simulink model "abssq06_fixpt16"  (R2021b)
settings: Solver=VariableStepAuto  StartTime=0.0  StopTime=99  RelTol=1e-3
undefined symbols (not defined in the file): S, vsva2197, xcvc1902
libraries: hdlBasic x65, vmcUtilities x1
settings Model: Creator=abeshu  LastModifiedBy=shu_abe

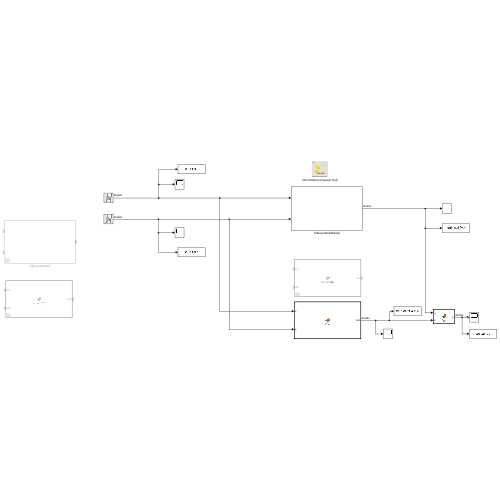
[thumbnail: Simulink's stored preview of the top-level diagram]
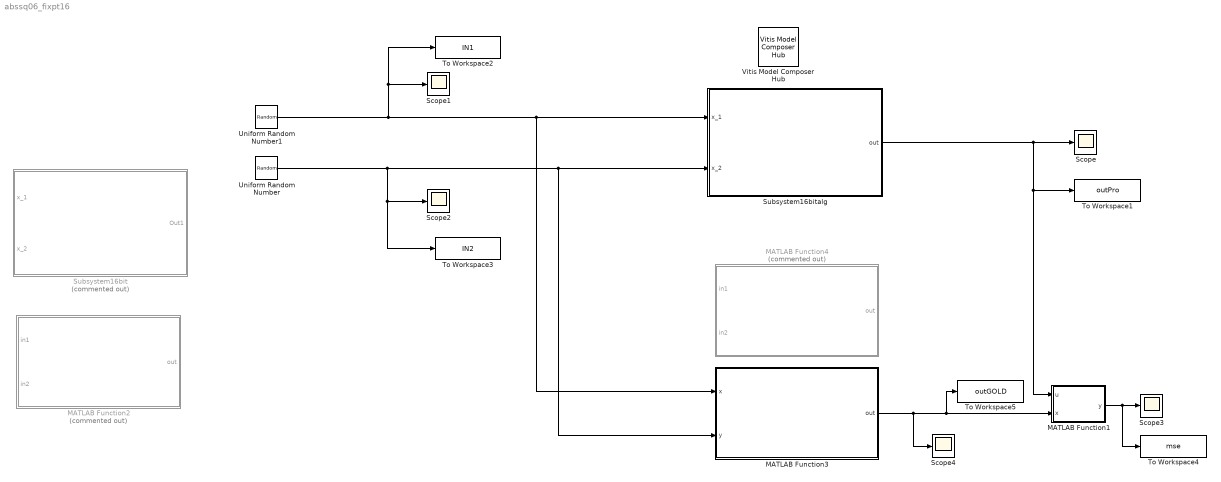
== system abssq06_fixpt16 ==
  MATLAB Function1 : MATLAB Function  TreatAsAtomicUnit=on
  MATLAB Function2 : MATLAB Function  Commented=on  TreatAsAtomicUnit=on
  MATLAB Function3 : MATLAB Function  TreatAsAtomicUnit=on
  MATLAB Function4 : MATLAB Function  Commented=on  TreatAsAtomicUnit=on
  Scope{,1..4} (5 alike) : Scope
  Subsystem16bit : Subsystem  Commented=on
      mask Display: %%%%
  Subsystem16bitalg : Subsystem
      mask Display: %%%%
  To Workspace1 : ToWorkspace  VariableName=outPro  SaveFormat=Structure With Time  SampleTime=-1
  To Workspace2 : ToWorkspace  VariableName=IN1  SaveFormat=Structure With Time  SampleTime=-1
  To Workspace3 : ToWorkspace  VariableName=IN2  SaveFormat=Structure With Time  SampleTime=-1
  To Workspace4 : ToWorkspace  VariableName=mse  SaveFormat=Structure With Time  SampleTime=-1
  To Workspace5 : ToWorkspace  VariableName=outGOLD  SaveFormat=Structure With Time  SampleTime=-1
  Uniform Random Number : UniformRandomNumber  SampleTime=1
  Uniform Random Number1 : UniformRandomNumber  Seed=1  SampleTime=1
  Vitis Model Composer Hub : vmcUtilities/Vitis Model Composer Hub  Tag=genX  CodeGeneration=off  SubsystemName=<enter or select subsystem name>  TargetDirectory=./code  ExportType=HLS C++ code  IpVendor=xilinx.com  IpLibrary=hls  IpVersion=1.0  IpHWLanguage=Verilog  AieCompilerOptions={}  CreateTestbench=off  TestbenchStackSize=10  RunAieSim=off  AieSimTimeout=50000  RunAieSimProfiling=off  LaunchVitisAnalyzer=off  PlotOutput=off  RunX86Sim=off  X86SimTimeout=10  GenHwImage=off  PlatformType=Not Specified  HwSystemType=Baremetal  HwValidationTarget=hw  ProjDevice=Alveo U250 Data Center Accelerator Card (xcu250-figd2104-2L-e)  ProjDevicePart=xcvc1902-vsva2197-2MP-e-S  SamplePeriod=-1  ClockFrequency=200  DataPathParallelism=1  xilinxfamily=virtexuplus  part=xcu250  speed=-2L-e  package=figd2104  directory=./abssq06alg_sim16  testbench=on  incr_netlist=off  synthesis_tool=Vivado  clock_wrapper=Clock Enables  dbl_ovrd=According to Block Masks  dcm_input_clock_period=10  sysclk_period=50  simulink_period=1  eval_field=0
  wires:
  Subsystem16bitalg/1(out) -> Scope/1, MATLAB Function1/1(u), To Workspace1/1
  MATLAB Function1/1(y) -> To Workspace4/1, Scope3/1
  MATLAB Function3/1(out) -> Scope4/1, To Workspace5/1, MATLAB Function1/2(x)
  Uniform Random Number1/1 -> Subsystem16bitalg/1(x_1), MATLAB Function3/1(x), To Workspace2/1, Scope1/1
  Uniform Random Number/1 -> Subsystem16bitalg/2(x_2), MATLAB Function3/2(y), To Workspace3/1, Scope2/1

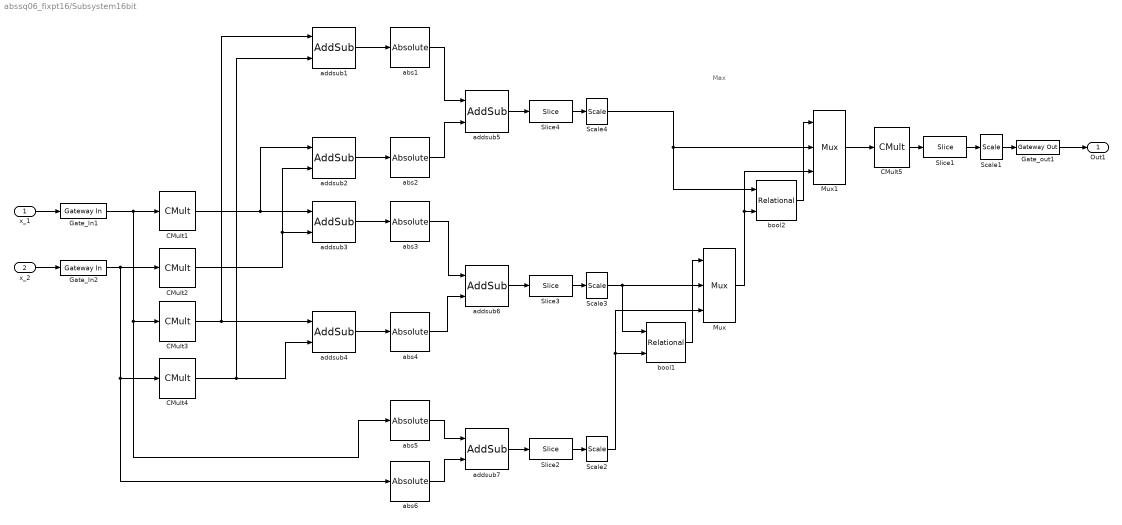
== system abssq06_fixpt16/Subsystem16bit ==
  note: Max
  x_1 : Inport
  x_2 : Inport  Port=2
  CMult1 : hdlBasic/CMult  const=cos(pi/6)  gui_display_data_type=Fixed-point  const_n_bits=16  const_bin_pt=15  float_type=Single  exp_bits=8  fraction_bits=24  en=off  latency=0  precision=Full  arith_type="Signed  (2's comp)"  n_bits=16  bin_pt=14  quantization=Truncate  overflow=Wrap  use_behavioral_HDL=off  mem_type=Distributed RAM  pipeline=off  XmcBlockStatus=1  maskContainerNames=tabcontainer1  block_type=cmult  block_config=sysgen:CMult_config
      settings: infoedit=[]
  CMult2 : hdlBasic/CMult  const=sin(pi/6)  gui_display_data_type=Fixed-point  const_n_bits=16  const_bin_pt=15  float_type=Single  exp_bits=8  fraction_bits=24  en=off  latency=0  precision=Full  arith_type="Signed  (2's comp)"  n_bits=16  bin_pt=14  quantization=Truncate  overflow=Wrap  use_behavioral_HDL=off  mem_type=Distributed RAM  pipeline=off  XmcBlockStatus=1  maskContainerNames=tabcontainer1  block_type=cmult  block_config=sysgen:CMult_config
      settings: infoedit=[]
  CMult3 : hdlBasic/CMult  const=sin(pi/6)  gui_display_data_type=Fixed-point  const_n_bits=16  const_bin_pt=15  float_type=Single  exp_bits=8  fraction_bits=24  en=off  latency=0  precision=Full  arith_type="Signed  (2's comp)"  n_bits=16  bin_pt=14  quantization=Truncate  overflow=Wrap  use_behavioral_HDL=off  mem_type=Distributed RAM  pipeline=off  XmcBlockStatus=1  maskContainerNames=tabcontainer1  block_type=cmult  block_config=sysgen:CMult_config
      settings: infoedit=[]
  CMult4 : hdlBasic/CMult  const=cos(pi/6)  gui_display_data_type=Fixed-point  const_n_bits=16  const_bin_pt=15  float_type=Single  exp_bits=8  fraction_bits=24  en=off  latency=0  precision=Full  arith_type="Signed  (2's comp)"  n_bits=16  bin_pt=14  quantization=Truncate  overflow=Wrap  use_behavioral_HDL=off  mem_type=Distributed RAM  pipeline=off  XmcBlockStatus=1  maskContainerNames=tabcontainer1  block_type=cmult  block_config=sysgen:CMult_config
      settings: infoedit=[]
  CMult5 : hdlBasic/CMult  const=1/sqrt(2)  gui_display_data_type=Fixed-point  const_n_bits=16  const_bin_pt=15  float_type=Single  exp_bits=8  fraction_bits=24  en=off  latency=0  precision=Full  arith_type="Signed  (2's comp)"  n_bits=16  bin_pt=14  quantization=Truncate  overflow=Wrap  use_behavioral_HDL=off  mem_type=Distributed RAM  pipeline=off  XmcBlockStatus=1  maskContainerNames=tabcontainer1  block_type=cmult  block_config=sysgen:CMult_config
      settings: infoedit=[]
  Gate_In1 : hdlBasic/Gateway In  gui_display_data_type=Fixed-point  arith_type=Signed (2's comp)  n_bits=16  bin_pt=14  preci_type=Double  exp_width=8  frac_width=24  rows=1  columns=1  quantization="Round  (unbiased: +/- Inf)"  overflow=Saturate  period=1  UseAsADC=off  ADCChannel='1'  interface=None  automatic_assignment=on  address_offset=hex2dec('00')  intf_name=''  intf_description=''  default_value=0  timing_constraint=None  locs_specified=off  LOCs={}  io_standard={}  inherit_from_input=off  hdl_port=on  XmcBlockStatus=1  maskContainerNames=group4  block_type=gatewayin  block_config=sysgen:gateway_in_config  block_width_w=590  block_height_w=620  block_width=640  block_height=850
  Gate_In2 : hdlBasic/Gateway In  gui_display_data_type=Fixed-point  arith_type=Signed (2's comp)  n_bits=16  bin_pt=14  preci_type=Double  exp_width=8  frac_width=24  rows=1  columns=1  quantization="Round  (unbiased: +/- Inf)"  overflow=Saturate  period=1  UseAsADC=off  ADCChannel='1'  interface=None  automatic_assignment=on  address_offset=hex2dec('00')  intf_name=''  intf_description=''  default_value=0  timing_constraint=None  locs_specified=off  LOCs={}  io_standard={}  inherit_from_input=off  hdl_port=on  XmcBlockStatus=1  maskContainerNames=group4  block_type=gatewayin  block_config=sysgen:gateway_in_config  block_width_w=590  block_height_w=620  block_width=640  block_height=850
  Gate_out1 : hdlBasic/Gateway Out  inherit_from_input=off  hdl_port=on  rows=1  columns=1  UseAsDAC=off  DACChannel='1'  interface=None  automatic_assignment=on  address_offset=hex2dec('00')  intf_name=''  intf_description=''  timing_constraint=None  locs_specified=off  LOCs={}  io_standard={}  XmcBlockStatus=1  maskContainerNames=group4  block_type=gatewayout  block_config=sysgen:gateway_out_config  block_width_w=590  block_height_w=620  block_width=620  block_height=750
  Mux : hdlBasic/Mux  inputs=2  en=off  latency=0  precision=Full  arith_type=Unsigned  n_bits=16  bin_pt=14  quantization=Truncate  overflow=Wrap  XmcBlockStatus=1  maskContainerNames=tabcontainer1  block_type=mux  block_config=sysgen:Mux_config
  Mux1 : hdlBasic/Mux  inputs=2  en=off  latency=0  precision=Full  arith_type=Unsigned  n_bits=16  bin_pt=14  quantization=Truncate  overflow=Wrap  XmcBlockStatus=1  maskContainerNames=tabcontainer1  block_type=mux  block_config=sysgen:Mux_config
  Scale1 : hdlBasic/Scale  scale_factor=-15  XmcBlockStatus=1  maskContainerNames=group1  block_type=scale  block_config=sysgen:Scale_config
  Scale2 : hdlBasic/Scale  scale_factor=-14  XmcBlockStatus=1  maskContainerNames=group1  block_type=scale  block_config=sysgen:Scale_config
  Scale3 : hdlBasic/Scale  scale_factor=-15  XmcBlockStatus=1  maskContainerNames=group1  block_type=scale  block_config=sysgen:Scale_config
  Scale4 : hdlBasic/Scale  scale_factor=-15  XmcBlockStatus=1  maskContainerNames=group1  block_type=scale  block_config=sysgen:Scale_config
  Slice1 : hdlBasic/Slice  nbits=8  boolean_output=off  mode=Two Bit Locations  bit1=-1  base1=MSB of Input  bit0=15  base0=LSB of Input  XmcBlockStatus=1  maskContainerNames=group1  block_type=slice  block_config=sysgen:Slice_config
  Slice2 : hdlBasic/Slice  nbits=15  boolean_output=off  mode=Upper Bit Location + Width  bit1=-3  base1=MSB of Input  bit0=7  base0=LSB of Input  XmcBlockStatus=1  maskContainerNames=group1  block_type=slice  block_config=sysgen:Slice_config
  Slice3 : hdlBasic/Slice  nbits=7  boolean_output=off  mode=Two Bit Locations  bit1=-5  base1=MSB of Input  bit0=14  base0=LSB of Input  XmcBlockStatus=1  maskContainerNames=group1  block_type=slice  block_config=sysgen:Slice_config
  Slice4 : hdlBasic/Slice  nbits=7  boolean_output=off  mode=Two Bit Locations  bit1=-5  base1=MSB of Input  bit0=14  base0=LSB of Input  XmcBlockStatus=1  maskContainerNames=group1  block_type=slice  block_config=sysgen:Slice_config
  abs{1..6} (6 alike) : hdlBasic/Absolute  precision=Full  arith_type=Unsigned  n_bits=16  bin_pt=14  quantization=Truncate  overflow=Wrap  en=off  latency=0  XmcBlockStatus=1  maskContainerNames=tabcontainer1  block_type=abs  block_config=sysgen:Abs_config
  addsub1 : hdlBasic/AddSub  mode=Subtraction  use_carryin=off  use_carryout=off  en=off  latency=0  precision=Full  arith_type="Signed  (2's comp)"  n_bits=35  bin_pt=32  quantization="Round  (unbiased: +/- Inf)"  overflow=Saturate  use_behavioral_HDL=off  hw_selection=Fabric  pipelined=on  XmcBlockStatus=1  maskContainerNames=tabcontainer1  block_type=addsub  block_config=sysgen:Addsub_config
  addsub{2,4..6} (4 alike) : hdlBasic/AddSub  mode=Addition  use_carryin=off  use_carryout=off  en=off  latency=0  precision=Full  arith_type=Unsigned  n_bits=16  bin_pt=14  quantization="Round  (unbiased: +/- Inf)"  overflow=Saturate  use_behavioral_HDL=off  hw_selection=Fabric  pipelined=on  XmcBlockStatus=1  maskContainerNames=tabcontainer1  block_type=addsub  block_config=sysgen:Addsub_config
  addsub3 : hdlBasic/AddSub  mode=Subtraction  use_carryin=off  use_carryout=off  en=off  latency=0  precision=Full  arith_type="Signed  (2's comp)"  n_bits=35  bin_pt=32  quantization="Round  (unbiased: +/- Inf)"  overflow=Saturate  use_behavioral_HDL=off  hw_selection=Fabric  pipelined=on  XmcBlockStatus=1  maskContainerNames=tabcontainer1  block_type=addsub  block_config=sysgen:Addsub_config
  addsub7 : hdlBasic/AddSub  mode=Addition  use_carryin=off  use_carryout=off  en=off  latency=0  precision=Full  arith_type=Unsigned  n_bits=17  bin_pt=16  quantization="Round  (unbiased: +/- Inf)"  overflow=Saturate  use_behavioral_HDL=off  hw_selection=Fabric  pipelined=on  XmcBlockStatus=1  maskContainerNames=tabcontainer1  block_type=addsub  block_config=sysgen:Addsub_config
  bool1 : hdlBasic/Relational  mode=a<b  op_type=Bool  en=off  latency=0  XmcBlockStatus=1  maskContainerNames=tabcontainer1  block_type=relational  block_config=sysgen:Relational_config
  bool2 : hdlBasic/Relational  mode=a<b  op_type=Bool  en=off  latency=0  XmcBlockStatus=1  maskContainerNames=tabcontainer1  block_type=relational  block_config=sysgen:Relational_config
  Out1 : Outport
  wires:
  addsub3/1 -> abs3/1
  abs3/1 -> addsub6/1
  CMult1/1 -> addsub3/1, addsub2/1
  CMult2/1 -> addsub3/2, addsub2/2
  CMult5/1 -> Slice1/1
  x_2/1 -> Gate_In2/1
  x_1/1 -> Gate_In1/1
  bool1/1 -> Mux/1
  addsub4/1 -> abs4/1
  abs4/1 -> addsub6/2
  Gate_In1/1 -> CMult1/1, abs5/1, CMult3/1
  Gate_In2/1 -> CMult4/1, abs6/1, CMult2/1
  CMult3/1 -> addsub4/1, addsub1/1
  CMult4/1 -> addsub4/2, addsub1/2
  addsub2/1 -> abs2/1
  abs2/1 -> addsub5/2
  addsub1/1 -> abs1/1
  abs1/1 -> addsub5/1
  Gate_out1/1 -> Out1/1
  Scale4/1 -> bool2/1, Mux1/2
  Mux/1 -> Mux1/3, bool2/2
  bool2/1 -> Mux1/1
  Mux1/1 -> CMult5/1
  abs5/1 -> addsub7/1
  abs6/1 -> addsub7/2
  Scale1/1 -> Gate_out1/1
  Slice1/1 -> Scale1/1
  addsub5/1 -> Slice4/1
  Slice3/1 -> Scale3/1
  Slice4/1 -> Scale4/1
  Slice2/1 -> Scale2/1
  addsub6/1 -> Slice3/1
  Scale3/1 -> Mux/2, bool1/1
  addsub7/1 -> Slice2/1
  Scale2/1 -> Mux/3, bool1/2

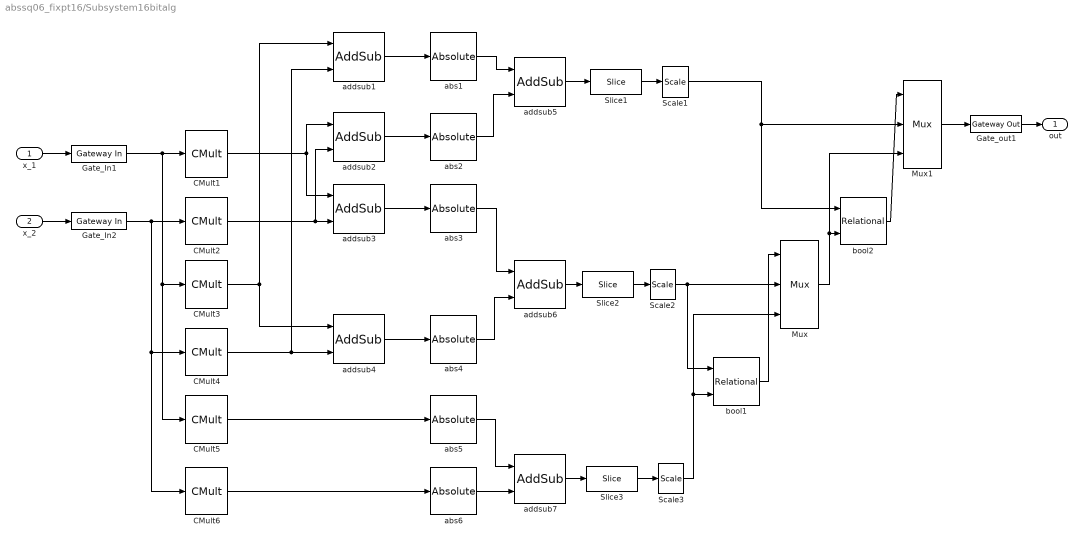
== system abssq06_fixpt16/Subsystem16bitalg ==
  x_1 : Inport
  x_2 : Inport  Port=2
  CMult1 : hdlBasic/CMult  const=1/sqrt(2)*cos(pi/6)  gui_display_data_type=Fixed-point  const_n_bits=16  const_bin_pt=15  float_type=Double  exp_bits=8  fraction_bits=24  en=off  latency=0  precision=Full  arith_type="Signed  (2's comp)"  n_bits=16  bin_pt=14  quantization=Truncate  overflow=Wrap  use_behavioral_HDL=off  mem_type=Distributed RAM  pipeline=off  XmcBlockStatus=1  maskContainerNames=tabcontainer1  block_type=cmult  block_config=sysgen:CMult_config
      settings: infoedit=[]
  CMult2 : hdlBasic/CMult  const=1/sqrt(2)*sin(pi/6)  gui_display_data_type=Fixed-point  const_n_bits=16  const_bin_pt=15  float_type=Double  exp_bits=8  fraction_bits=24  en=off  latency=0  precision=Full  arith_type="Signed  (2's comp)"  n_bits=16  bin_pt=14  quantization=Truncate  overflow=Wrap  use_behavioral_HDL=off  mem_type=Distributed RAM  pipeline=off  XmcBlockStatus=1  maskContainerNames=tabcontainer1  block_type=cmult  block_config=sysgen:CMult_config
      settings: infoedit=[]
  CMult3 : hdlBasic/CMult  const=1/sqrt(2)*sin(pi/6)  gui_display_data_type=Fixed-point  const_n_bits=16  const_bin_pt=15  float_type=Double  exp_bits=8  fraction_bits=24  en=off  latency=0  precision=Full  arith_type="Signed  (2's comp)"  n_bits=16  bin_pt=14  quantization=Truncate  overflow=Wrap  use_behavioral_HDL=off  mem_type=Distributed RAM  pipeline=off  XmcBlockStatus=1  maskContainerNames=tabcontainer1  block_type=cmult  block_config=sysgen:CMult_config
      settings: infoedit=[]
  CMult4 : hdlBasic/CMult  const=1/sqrt(2)*cos(pi/6)  gui_display_data_type=Fixed-point  const_n_bits=16  const_bin_pt=15  float_type=Double  exp_bits=8  fraction_bits=24  en=off  latency=0  precision=Full  arith_type="Signed  (2's comp)"  n_bits=16  bin_pt=14  quantization=Truncate  overflow=Wrap  use_behavioral_HDL=off  mem_type=Distributed RAM  pipeline=off  XmcBlockStatus=1  maskContainerNames=tabcontainer1  block_type=cmult  block_config=sysgen:CMult_config
      settings: infoedit=[]
  CMult5 : hdlBasic/CMult  const=1/sqrt(2)  gui_display_data_type=Fixed-point  const_n_bits=16  const_bin_pt=15  float_type=Double  exp_bits=8  fraction_bits=24  en=off  latency=0  precision=Full  arith_type="Signed  (2's comp)"  n_bits=16  bin_pt=14  quantization=Truncate  overflow=Wrap  use_behavioral_HDL=off  mem_type=Distributed RAM  pipeline=off  XmcBlockStatus=1  maskContainerNames=tabcontainer1  block_type=cmult  block_config=sysgen:CMult_config
      settings: infoedit=[]
  CMult6 : hdlBasic/CMult  const=1/sqrt(2)  gui_display_data_type=Fixed-point  const_n_bits=16  const_bin_pt=15  float_type=Double  exp_bits=8  fraction_bits=24  en=off  latency=0  precision=Full  arith_type="Signed  (2's comp)"  n_bits=16  bin_pt=14  quantization=Truncate  overflow=Wrap  use_behavioral_HDL=off  mem_type=Distributed RAM  pipeline=off  XmcBlockStatus=1  maskContainerNames=tabcontainer1  block_type=cmult  block_config=sysgen:CMult_config
      settings: infoedit=[]
  Gate_In1 : hdlBasic/Gateway In  gui_display_data_type=Fixed-point  arith_type=Signed (2's comp)  n_bits=16  bin_pt=14  preci_type=Double  exp_width=8  frac_width=24  rows=1  columns=1  quantization="Round  (unbiased: +/- Inf)"  overflow=Saturate  period=1  UseAsADC=off  ADCChannel='1'  interface=None  automatic_assignment=on  address_offset=hex2dec('00')  intf_name=''  intf_description=''  default_value=0  timing_constraint=None  locs_specified=off  LOCs={}  io_standard={}  inherit_from_input=off  hdl_port=on  XmcBlockStatus=1  maskContainerNames=group4  block_type=gatewayin  block_config=sysgen:gateway_in_config  block_width_w=590  block_height_w=620  block_width=640  block_height=850
  Gate_In2 : hdlBasic/Gateway In  gui_display_data_type=Fixed-point  arith_type=Signed (2's comp)  n_bits=16  bin_pt=14  preci_type=Double  exp_width=8  frac_width=24  rows=1  columns=1  quantization="Round  (unbiased: +/- Inf)"  overflow=Saturate  period=1  UseAsADC=off  ADCChannel='1'  interface=None  automatic_assignment=on  address_offset=hex2dec('00')  intf_name=''  intf_description=''  default_value=0  timing_constraint=None  locs_specified=off  LOCs={}  io_standard={}  inherit_from_input=off  hdl_port=on  XmcBlockStatus=1  maskContainerNames=group4  block_type=gatewayin  block_config=sysgen:gateway_in_config  block_width_w=590  block_height_w=620  block_width=640  block_height=850
  Gate_out1 : hdlBasic/Gateway Out  inherit_from_input=off  hdl_port=on  rows=1  columns=1  UseAsDAC=off  DACChannel='1'  interface=None  automatic_assignment=on  address_offset=hex2dec('00')  intf_name=''  intf_description=''  timing_constraint=None  locs_specified=off  LOCs={}  io_standard={}  XmcBlockStatus=1  maskContainerNames=group4  block_type=gatewayout  block_config=sysgen:gateway_out_config  block_width_w=590  block_height_w=620  block_width=620  block_height=750
  Mux : hdlBasic/Mux  inputs=2  en=off  latency=0  precision=Full  arith_type=Unsigned  n_bits=16  bin_pt=14  quantization=Truncate  overflow=Wrap  XmcBlockStatus=1  maskContainerNames=tabcontainer1  block_type=mux  block_config=sysgen:Mux_config
  Mux1 : hdlBasic/Mux  inputs=2  en=off  latency=0  precision=Full  arith_type=Unsigned  n_bits=16  bin_pt=14  quantization=Truncate  overflow=Wrap  XmcBlockStatus=1  maskContainerNames=tabcontainer1  block_type=mux  block_config=sysgen:Mux_config
  Scale1 : hdlBasic/Scale  scale_factor=-15  XmcBlockStatus=1  maskContainerNames=group1  block_type=scale  block_config=sysgen:Scale_config
  Scale2 : hdlBasic/Scale  scale_factor=-15  XmcBlockStatus=1  maskContainerNames=group1  block_type=scale  block_config=sysgen:Scale_config
  Scale3 : hdlBasic/Scale  scale_factor=-15  XmcBlockStatus=1  maskContainerNames=group1  block_type=scale  block_config=sysgen:Scale_config
  Slice1 : hdlBasic/Slice  nbits=7  boolean_output=off  mode=Two Bit Locations  bit1=-5  base1=MSB of Input  bit0=14  base0=LSB of Input  XmcBlockStatus=1  maskContainerNames=group1  block_type=slice  block_config=sysgen:Slice_config
  Slice2 : hdlBasic/Slice  nbits=7  boolean_output=off  mode=Two Bit Locations  bit1=-5  base1=MSB of Input  bit0=14  base0=LSB of Input  XmcBlockStatus=1  maskContainerNames=group1  block_type=slice  block_config=sysgen:Slice_config
  Slice3 : hdlBasic/Slice  nbits=16  boolean_output=off  mode=Upper Bit Location + Width  bit1=-4  base1=MSB of Input  bit0=7  base0=LSB of Input  XmcBlockStatus=1  maskContainerNames=group1  block_type=slice  block_config=sysgen:Slice_config
  abs{1..6} (6 alike) : hdlBasic/Absolute  precision=Full  arith_type=Unsigned  n_bits=16  bin_pt=14  quantization=Truncate  overflow=Wrap  en=off  latency=0  XmcBlockStatus=1  maskContainerNames=tabcontainer1  block_type=abs  block_config=sysgen:Abs_config
  addsub1 : hdlBasic/AddSub  mode=Subtraction  use_carryin=off  use_carryout=off  en=off  latency=0  precision=Full  arith_type="Signed  (2's comp)"  n_bits=35  bin_pt=32  quantization="Round  (unbiased: +/- Inf)"  overflow=Saturate  use_behavioral_HDL=off  hw_selection=Fabric  pipelined=on  XmcBlockStatus=1  maskContainerNames=tabcontainer1  block_type=addsub  block_config=sysgen:Addsub_config
  addsub{2,4..6} (4 alike) : hdlBasic/AddSub  mode=Addition  use_carryin=off  use_carryout=off  en=off  latency=0  precision=Full  arith_type=Unsigned  n_bits=16  bin_pt=14  quantization="Round  (unbiased: +/- Inf)"  overflow=Saturate  use_behavioral_HDL=off  hw_selection=Fabric  pipelined=on  XmcBlockStatus=1  maskContainerNames=tabcontainer1  block_type=addsub  block_config=sysgen:Addsub_config
  addsub3 : hdlBasic/AddSub  mode=Subtraction  use_carryin=off  use_carryout=off  en=off  latency=0  precision=Full  arith_type="Signed  (2's comp)"  n_bits=35  bin_pt=32  quantization="Round  (unbiased: +/- Inf)"  overflow=Saturate  use_behavioral_HDL=off  hw_selection=Fabric  pipelined=on  XmcBlockStatus=1  maskContainerNames=tabcontainer1  block_type=addsub  block_config=sysgen:Addsub_config
  addsub7 : hdlBasic/AddSub  mode=Addition  use_carryin=off  use_carryout=off  en=off  latency=0  precision=Full  arith_type=Unsigned  n_bits=17  bin_pt=16  quantization="Round  (unbiased: +/- Inf)"  overflow=Saturate  use_behavioral_HDL=off  hw_selection=Fabric  pipelined=on  XmcBlockStatus=1  maskContainerNames=tabcontainer1  block_type=addsub  block_config=sysgen:Addsub_config
  bool1 : hdlBasic/Relational  mode=a<b  op_type=Bool  en=off  latency=0  XmcBlockStatus=1  maskContainerNames=tabcontainer1  block_type=relational  block_config=sysgen:Relational_config
  bool2 : hdlBasic/Relational  mode=a<b  op_type=Bool  en=off  latency=0  XmcBlockStatus=1  maskContainerNames=tabcontainer1  block_type=relational  block_config=sysgen:Relational_config
  out : Outport
  wires:
  addsub3/1 -> abs3/1
  abs3/1 -> addsub6/1
  CMult1/1 -> addsub3/1, addsub2/1
  CMult2/1 -> addsub3/2, addsub2/2
  x_2/1 -> Gate_In2/1
  x_1/1 -> Gate_In1/1
  bool1/1 -> Mux/1
  addsub4/1 -> abs4/1
  abs4/1 -> addsub6/2
  Gate_In1/1 -> CMult1/1, CMult5/1, CMult3/1
  Gate_In2/1 -> CMult4/1, CMult6/1, CMult2/1
  CMult3/1 -> addsub4/1, addsub1/1
  CMult4/1 -> addsub4/2, addsub1/2
  addsub2/1 -> abs2/1
  abs2/1 -> addsub5/2
  addsub1/1 -> abs1/1
  abs1/1 -> addsub5/1
  Gate_out1/1 -> out/1
  Scale1/1 -> bool2/1, Mux1/2
  Mux/1 -> Mux1/3, bool2/2
  bool2/1 -> Mux1/1
  abs5/1 -> addsub7/1
  abs6/1 -> addsub7/2
  Mux1/1 -> Gate_out1/1
  Slice2/1 -> Scale2/1
  Slice1/1 -> Scale1/1
  Slice3/1 -> Scale3/1
  Scale2/1 -> bool1/1, Mux/2
  Scale3/1 -> Mux/3, bool1/2
  CMult5/1 -> abs5/1
  CMult6/1 -> abs6/1
  addsub5/1 -> Slice1/1
  addsub6/1 -> Slice2/1
  addsub7/1 -> Slice3/1

== matlab function abssq06_fixpt16/MATLAB Function2 ==
  data: in1 input; out output; in2 input
function out = abssq06(in1,in2)

SIN_PI_6 = sin(pi/6);
SIN_2PI_6 = sin(2*pi/6);
COS_PI_6 = cos(pi/6);
COS_2PI_6 = cos(2*pi/6);

% Real and imaginary part


% theta = 0
a0 = abs(in1) + abs(in2);
% theta = pi/4
%a1 = abs(COS_PI_4*in1 - SIN_PI_4*in2) ...
%    + abs(SIN_PI_4*in1 + COS_PI_4*in2);

% theta = pi/6
a1 = abs(COS_PI_6*in1 - SIN_PI_6*in2) + abs(SIN_PI_6*in1 + COS_PI_6*in2);
% theta = 2pi/6
a2 = abs(COS_2PI_6*in1 - SIN_2PI_6*in2) + abs(SIN_2PI_6*in1 + COS_2PI_6*in2);


out = (1/sqrt(2)).*max(max(a0, a1),a2);

end

== matlab function abssq06_fixpt16/MATLAB Function3 ==
  data: x input; out output; y input
function out = fcn(x,y)
out = sqrt(x.^2 + y.^2);

== matlab function abssq06_fixpt16/MATLAB Function4 ==
  data: in1 input; out output; in2 input
function out = abssq06(in1,in2)

SQRT_2 = 1/sqrt(2);
SIN_PI_6 = SQRT_2*sin(pi/6);
SIN_2PI_6 = SQRT_2*sin(2*pi/6);
COS_PI_6 = SQRT_2*cos(pi/6);
COS_2PI_6 = SQRT_2*cos(2*pi/6);

% Real and imaginary part


% theta = 0
a0 = abs(SQRT_2*in1) + abs(SQRT_2*in2);
% theta = pi/6
a1 = abs(COS_PI_6*in1 + SIN_PI_6*in2) + abs(SIN_PI_6*in1 - COS_PI_6*in2);
% theta = 2pi/6
a2 = abs(COS_2PI_6*in1 + SIN_2PI_6*in2) + abs(SIN_2PI_6*in1 - COS_2PI_6*in2);


out = max(max(a0, a1),a2);

end

== matlab function abssq06_fixpt16/MATLAB Function1 ==
  data: u input; y output; x input
function y = fcn(u,x)
y = immse(u,x);
